simulink model "combined_model"  (R2015a)
settings: Solver=ode4  StartTime=0  StopTime=1  FixedStep=0.0001  MaxStep=0.001  RelTol=1e-3
undefined symbols (not defined in the file): air_viscosity, car_speed, coil_turns, coil_wire_length, cylinder_area, cylinder_height, data, flux_linkage, magnet_diameter, magnet_height, magnet_mass, radial_clearance, tyre_pressure, tyre_radius, tyre_temperature
libraries: simulink x2
settings Model: Creator=ojousima  LastModifiedBy=ojousima
settings SolverCC: ZeroCrossControl=DisableAll  ZeroCrossAlgorithm=Adaptive

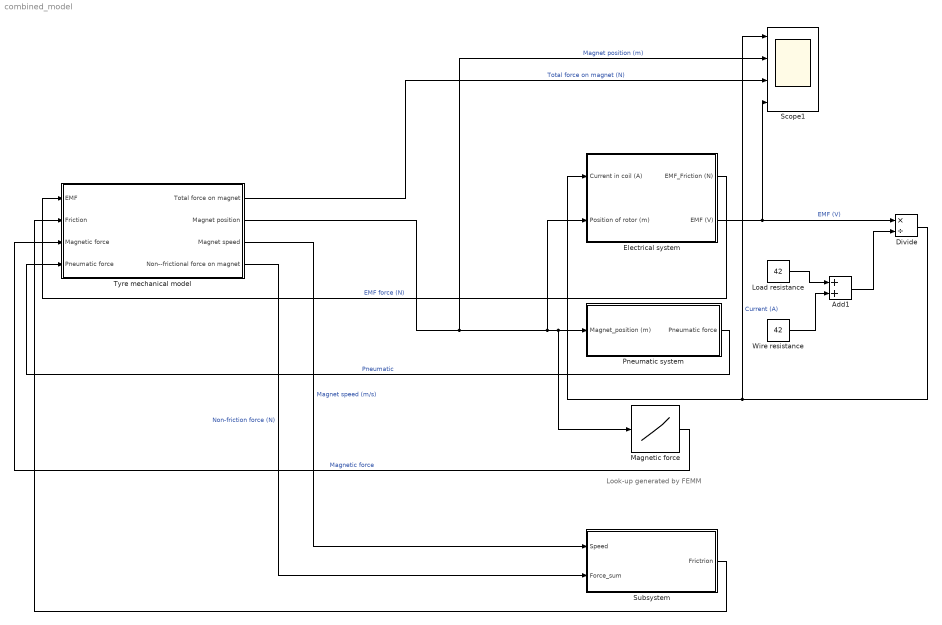
== system combined_model ==
  note: Look-up generated by FEMM
  Add1 : Sum
  Divide : Product  Inputs=*/
  Electrical system : Subsystem
  Load resistance : Constant  Value=42
  Magnetic force : Lookup_n-D  InitFcn=|  NumberOfTableDimensions=1  BreakpointsForDimension1=[-0.0087:0.0001:0.0086]  Table=data  ExtrapMethod=Clip  DiagnosticForOutOfRangeInput=Error  UseLastTableValue=on  InternalRulePriority=Speed  RndMeth=Simplest  InputSameDT=on
      | %Import the data from csv
      | data = csvread('force.csv');
      | data = data(:, 1);
  Pneumatic system : Subsystem
  Scope1 : Scope  NumInputPorts=4
      settings: YMin=-3.5~-1e-08~-4.5e-06~-0.0025  YMax=3~1e-09~1e-06~0.00175  SaveName=ScopeData2  MaxDataPoints=100000
  Subsystem : Subsystem
  Tyre mechanical model : Subsystem
  Wire resistance : Constant  Value=42
  wires:
  Electrical system/2(EMF (V)) -> Scope1/4, Divide/1  "EMF (V)"
  Load resistance/1 -> Add1/1
  Wire resistance/1 -> Add1/2
  Add1/1 -> Divide/2
  Divide/1 -> Scope1/1, Electrical system/1(Current in coil (A))  "Current (A)"
  Tyre mechanical model/2(Magnet position) -> Scope1/2, Electrical system/2(Position of rotor (m)), Magnetic force/1, Pneumatic system/1(Magnet_position (m))  "Magnet position (m)"
  Tyre mechanical model/3(Magnet speed) -> Subsystem/1(Speed)  "Magnet speed (m/s)"
  Tyre mechanical model/4(Non--frictional force on magnet) -> Subsystem/2(Force_sum)  "Non-friction force (N)"
  Magnetic force/1 -> Tyre mechanical model/3(Magnetic force)  "Magnetic force"
  Pneumatic system/1(Pneumatic force) -> Tyre mechanical model/4(Pneumatic force)  "Pneumatic"
  Electrical system/1(EMF_Friction (N)) -> Tyre mechanical model/1(EMF)  "EMF force (N)"
  Subsystem/1(Frictrion) -> Tyre mechanical model/2(Friction)
  Tyre mechanical model/1("Total force on magnet ") -> Scope1/3  "Total force on magnet (N)"

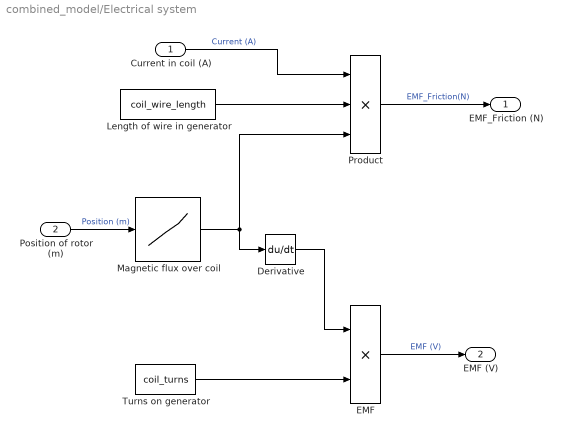
== system combined_model/Electrical system ==
  Current in coil (A) : Inport
  Position of rotor (m) : Inport  Port=2
  Derivative : Derivative
  EMF : Product
  Length of wire in generator : Constant  Value=coil_wire_length
  Magnetic flux over coil : Lookup_n-D  InitFcn=|  NumberOfTableDimensions=1  BreakpointsForDimension1=[-0.0087:0.0001:0.0086]  Table=flux_linkage  DiagnosticForOutOfRangeInput=Error  InternalRulePriority=Speed  RndMeth=Simplest  InputSameDT=on
      | %Import the data from csv
      | flux_linkage = csvread('linkage.csv');
      | flux_linkage = flux_linkage(:, 1);
  Product : Product  Inputs=3
  Turns on generator : Constant  Value=coil_turns
  EMF_Friction (N) : Outport
  EMF (V) : Outport  Port=2
  wires:
  Magnetic flux over coil/1 -> Product/3, Derivative/1
  Position of rotor (m)/1 -> Magnetic flux over coil/1  "Position (m)"
  Length of wire in generator/1 -> Product/2
  Turns on generator/1 -> EMF/2
  EMF/1 -> EMF (V)/1  "EMF (V)"
  Product/1 -> EMF_Friction (N)/1  "EMF_Friction(N)"
  Current in coil (A)/1 -> Product/1  "Current (A)"
  Derivative/1 -> EMF/1

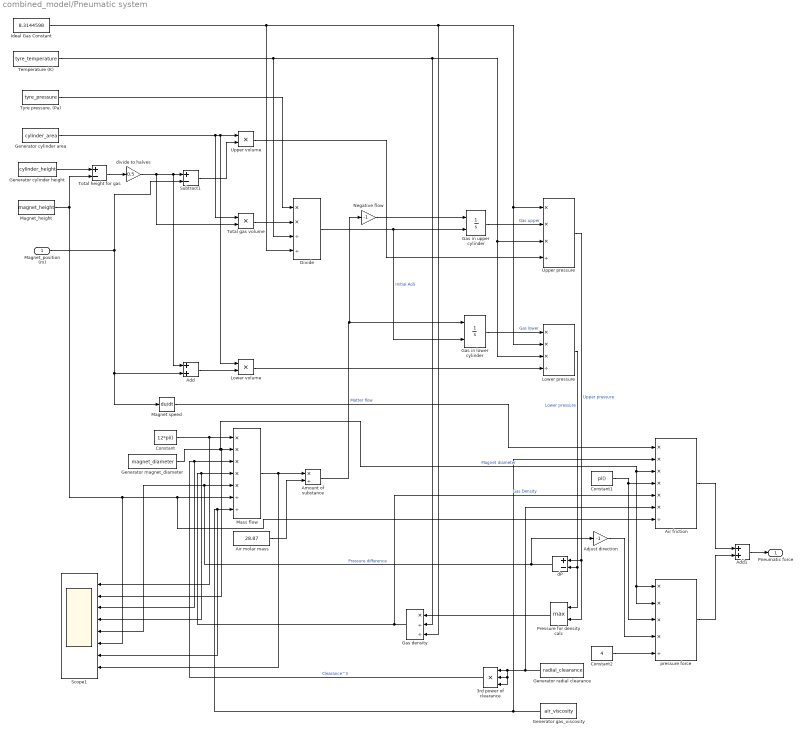
== system combined_model/Pneumatic system ==
  Magnet_position (m) : Inport
  3rd power of clearance : Product  Inputs=3
  Add : Sum
  Add1 : Sum
  Adjust direction : Gain  Gain=-1
  Air friction : Product  Inputs=******/
  Air molar mass : Constant  Value=28.87
  Amount of substance : Product  Inputs=*/
  Constant : Constant  Value=12*pi()
  Constant1 : Constant  Value=pi()
  Constant2 : Constant  Value=4
  Divide : Product  Inputs=**//
  Gas density : Product  Inputs=*//
  Gas in lower cylinder : Integrator  InitialConditionSource=external
  Gas in upper cylinder : Integrator  InitialConditionSource=external
  Generator cylinder area : Constant  Value=cylinder_area
  Generator cylinder height : Constant  Value=cylinder_height
  "Generator gas_viscosity " : Constant  Value=air_viscosity
  Generator magnet_diameter : Constant  Value=magnet_diameter
  Generator radial clearance : Constant  Value=radial_clearance
  Ideal Gas Constant : Constant  Value=8.3144598
  Lower pressure : Product  Inputs=***/
  Lower volume : Product
  Magnet speed : Derivative
  Magnet_height : Constant  Value=magnet_height
  Mass flow : Product  Inputs=*****//
  Negative flow : Gain  Gain=-1
  Pressure for density calc : MinMax  Function=max  Inputs=2
  Scope1 : Scope  NumInputPorts=8
      settings: YMin=37.6991~0.011~1.25e-10~80~-200000~0.00238~3.5~-0.15  YMax=37.6991~0.011~1.25e-10~150~250000~0.00238~3.5~0.25
  Subtract1 : Sum  Inputs=+-
  "Temperature (K) " : Constant  Value=tyre_temperature
  Total gas volume : Product
  Total height for gas : Sum  Inputs=+-
  "Tyre pressure, (Pa)" : Constant  Value=tyre_pressure
  Upper pressure : Product  Inputs=***/
  Upper volume : Product
  dP : Sum  Inputs=+-
  divide to halves : Gain  Gain=0.5
  pressure force : Product  Inputs=****/
  Pneumatic force : Outport
  wires:
  Gas in lower cylinder/1 -> Lower pressure/1  "Gas lower"
  Ideal Gas Constant/1 -> Divide/4, Gas density/3, Upper pressure/1, Lower pressure/2
  "Temperature (K) "/1 -> Divide/3, Gas density/2, Lower pressure/3, Upper pressure/3
  Generator cylinder height/1 -> Total height for gas/1
  Total height for gas/1 -> divide to halves/1
  divide to halves/1 -> Total gas volume/2, Add/1, Subtract1/1
  Generator cylinder area/1 -> Total gas volume/1, Lower volume/1, Upper volume/1
  Subtract1/1 -> Upper volume/2
  Upper volume/1 -> Upper pressure/4
  Add/1 -> Lower volume/2
  Lower volume/1 -> Lower pressure/4
  Gas in upper cylinder/1 -> Upper pressure/2  "Gas upper"
  "Tyre pressure, (Pa)"/1 -> Divide/1
  Total gas volume/1 -> Divide/2
  Divide/1 -> Gas in lower cylinder/2, Gas in upper cylinder/2  "Initial AoS"
  Upper pressure/1 -> Pressure for density calc/2, dP/1  "Upper pressure"
  Lower pressure/1 -> Pressure for density calc/1, dP/2  "Lower pressure"
  Pressure for density calc/1 -> Gas density/1
  Generator radial clearance/1 -> Air friction/6, 3rd power of clearance/3, 3rd power of clearance/2, 3rd power of clearance/1
  Constant/1 -> Scope1/1, Mass flow/1
  Mass flow/1 -> Scope1/8, Amount of substance/1
  Generator magnet_diameter/1 -> Scope1/2, Mass flow/2, pressure force/1, pressure force/2, Air friction/3  "Magnet diameter"
  Constant1/1 -> pressure force/3, Air friction/4
  dP/1 -> Adjust direction/1, Mass flow/5, Scope1/5  "Pressure difference"
  Adjust direction/1 -> pressure force/4
  Constant2/1 -> pressure force/5
  Magnet_position (m)/1 -> Add/2, Magnet speed/1, Subtract1/2
  Air molar mass/1 -> Amount of substance/2
  3rd power of clearance/1 -> Scope1/3, Mass flow/3  "Clearance^3"
  Gas density/1 -> Air friction/5, Scope1/4, Mass flow/4  "Gas Density"
  "Generator gas_viscosity "/1 -> Air friction/2, Scope1/7, Mass flow/7
  Amount of substance/1 -> Negative flow/1, Gas in lower cylinder/1  "Matter flow"
  Negative flow/1 -> Gas in upper cylinder/1
  Magnet speed/1 -> Air friction/1
  Magnet_height/1 -> Total height for gas/2, Scope1/6, Air friction/7, Mass flow/6
  Add1/1 -> Pneumatic force/1
  Air friction/1 -> Add1/1
  pressure force/1 -> Add1/2

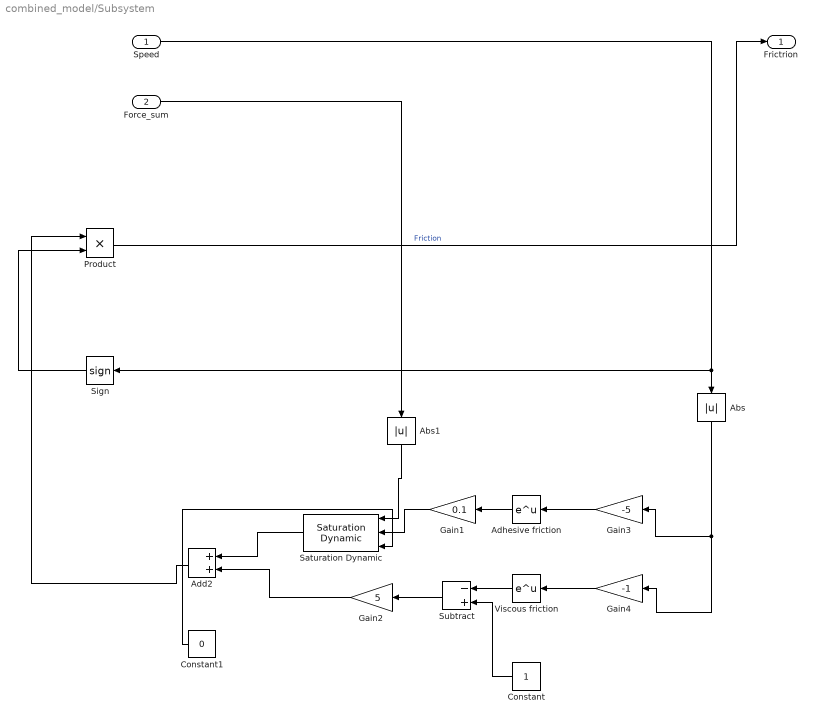
== system combined_model/Subsystem ==
  Speed : Inport
  Force_sum : Inport  Port=2
  Abs : Abs
  Abs1 : Abs
  Add2 : Sum
  Adhesive friction : Math  SaturateOnIntegerOverflow=on
  Constant : Constant
  Constant1 : Constant  Value=0
  Gain1 : Gain  Gain=0.1
  Gain2 : Gain  Gain=5
  Gain3 : Gain  Gain=-5
  Gain4 : Gain  Gain=-1
  Product : Product
  Saturation Dynamic : simulink/Discontinuities/Saturation Dynamic  OutMin=[]  OutMax=[]  OutDataTypeStr=Inherit: Same as second input  OutDataType=fixdt(1, 16)  OutScaling=2^-10  DoSatur=off
  Sign : Signum
  Subtract : Sum  Inputs=-+
  Viscous friction : Math  SaturateOnIntegerOverflow=on
  Frictrion : Outport
  wires:
  Adhesive friction/1 -> Gain1/1
  Gain3/1 -> Adhesive friction/1
  Gain4/1 -> Viscous friction/1
  Subtract/1 -> Gain2/1
  Viscous friction/1 -> Subtract/1
  Constant/1 -> Subtract/2
  Abs/1 -> Gain3/1, Gain4/1
  Sign/1 -> Product/2
  Constant1/1 -> Saturation Dynamic/3
  Gain1/1 -> Saturation Dynamic/2
  Saturation Dynamic/1 -> Add2/1
  Add2/1 -> Product/1
  Speed/1 -> Sign/1, Abs/1
  Force_sum/1 -> Abs1/1
  Product/1 -> Frictrion/1  "Friction"
  Gain2/1 -> Add2/2
  Abs1/1 -> Saturation Dynamic/1

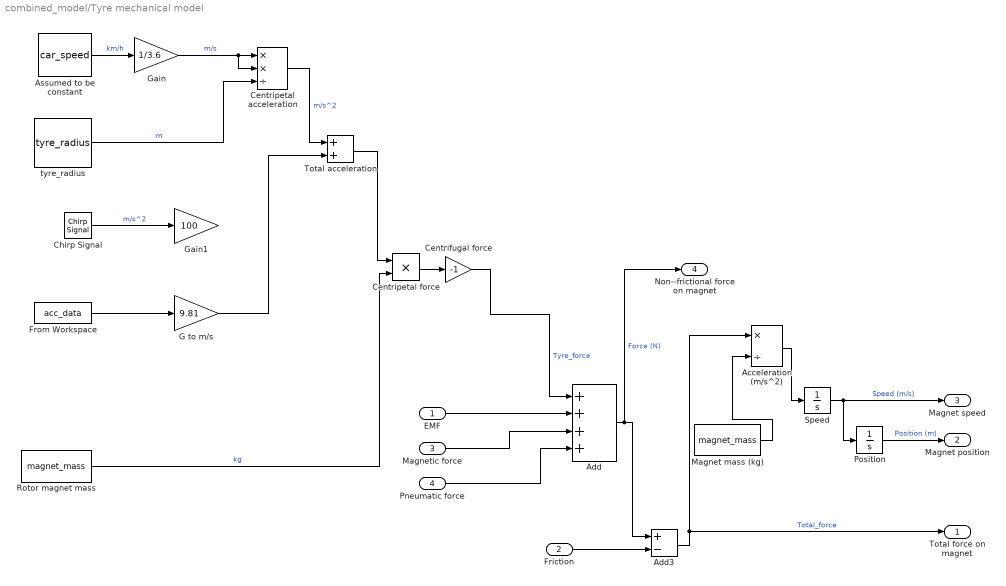
== system combined_model/Tyre mechanical model ==
  EMF : Inport
  Friction : Inport  Port=2
  Magnetic force : Inport  Port=3
  Pneumatic force : Inport  Port=4
  Acceleration (m/s^2) : Product  Inputs=*/
  Add : Sum  Inputs=++++
  Add3 : Sum  Inputs=+-
  Assumed to be constant : Constant  Value=car_speed
  Centrifugal force : Gain  Gain=-1
  Centripetal acceleration : Product  Inputs=**/
  Centripetal force : Product
  Chirp Signal : simulink/Sources/Chirp Signal  f1=10  T=10  f2=600
  From Workspace : FromWorkspace  VariableName=acc_data  SampleTime=0  OutputAfterFinalValue=Setting to zero
  G to m/s : Gain  Gain=9.81
  Gain : Gain  Gain=1/3.6
  Gain1 : Gain  Gain=100
  Magnet mass (kg) : Constant  Value=magnet_mass
  Position : Integrator
  Rotor magnet mass : Constant  Value=magnet_mass
  Speed : Integrator
  Total acceleration : Sum
  tyre_radius : Constant  Value=tyre_radius
  "Total force on magnet " : Outport
  Magnet position : Outport  Port=2
  Magnet speed : Outport  Port=3
  Non--frictional force on magnet : Outport  Port=4
  wires:
  Assumed to be constant/1 -> Gain/1  "km/h"
  Gain/1 -> Centripetal acceleration/2, Centripetal acceleration/1  "m/s"
  tyre_radius/1 -> Centripetal acceleration/3  "m"
  Centripetal acceleration/1 -> Total acceleration/1  "m/s^2"
  Chirp Signal/1 -> Gain1/1  "m/s^2"
  Total acceleration/1 -> Centripetal force/1
  Rotor magnet mass/1 -> Centripetal force/2  "kg"
  Centripetal force/1 -> Centrifugal force/1
  Centrifugal force/1 -> Add/1  "Tyre_force"
  Add/1 -> Non--frictional force on magnet/1, Add3/1  "Force (N)"
  Acceleration (m/s^2)/1 -> Speed/1
  Speed/1 -> Magnet speed/1, Position/1  "Speed (m/s)"
  Magnet mass (kg)/1 -> Acceleration (m/s^2)/2
  Add3/1 -> "Total force on magnet "/1, Acceleration (m/s^2)/1  "Total_force"
  Friction/1 -> Add3/2
  EMF/1 -> Add/2
  Magnetic force/1 -> Add/3
  Pneumatic force/1 -> Add/4
  Position/1 -> Magnet position/1  "Position (m)"
  From Workspace/1 -> G to m/s/1
  G to m/s/1 -> Total acceleration/2
